simulink model "Main_Sim"  (R2018a)
settings: Solver=ode1  StartTime=0.0  StopTime=constants.t_end  FixedStep=constants.dt  RelTol=1e-3  EnableMultiTasking=on
settings Model: ExtModeTrigDuration=5000  Creator=bruders  LastModifiedBy=Joseph
settings SolverCC: PositivePriorityOrder=on
settings DataIOCC: LimitDataPoints=on  SaveFormat=Array
settings OptimizationCC: LifeSpan=inf
settings DebuggingCC: SolverPrmCheckMsg=warning  AllowSymbolicDim=off  SFUnexpectedBacktrackingDiag=warning  SFNoUnconditionalDefaultTransitionDiag=warning  SFExecutionAtInitializationDiag=none
settings HardwareCC: ProdBitPerPointer=32  ProdBitPerSizeT=32  ProdBitPerPtrDiffT=32  ProdLargestAtomicFloat=None  ProdIntDivRoundTo=Undefined  ProdEndianess=Unspecified  ProdWordSize=32  ProdHWDeviceType=32-bit Generic
settings ModelReferenceCC: PropagateSignalLabelsOutOfModel=off
settings RTWCC: Description=QUARC Win64 Target  SystemTargetFile=quarc_win64.tlc  TemplateMakefile=quarc_default_tmf
settings CodeAppCC: StateflowObjectComments=on
settings STFCustomTargetCC: TargetPreCompLibLocation=C:\PROGRA~3\QUARC\lib\2016b\win64\release  ConcurrentExecutionCompliant=on  GeneratePreprocessorConditionals=Disable all  SystemTargetFile=quarc_win64.tlc
settings GRTTargetCC: TargetPreCompLibLocation=C:\PROGRA~3\QUARC\lib\2016b\win64\release  TargetLangStandard=C89/C90 (ANSI)  ParMdlRefBuildCompliant=off  CompOptLevelCompliant=off  GeneratePreprocessorConditionals=Disable all  CombineOutputUpdateFcns=off  MatFileLogging=off  CPPClassGenCompliant=off  GRTInterface=on  UseToolchainInfoCompliant=off  ExtMode=on  ExtModeMexFile=quarc_comm
settings ConfigComp: CovMetricSettings=dw  CovHtmlReporting=on  CovSaveCumulativeToWorkspaceVar=on  CovSaveSingleToWorkspaceVar=on  CovExternalEMLEnable=off  CovSFcnEnable=off

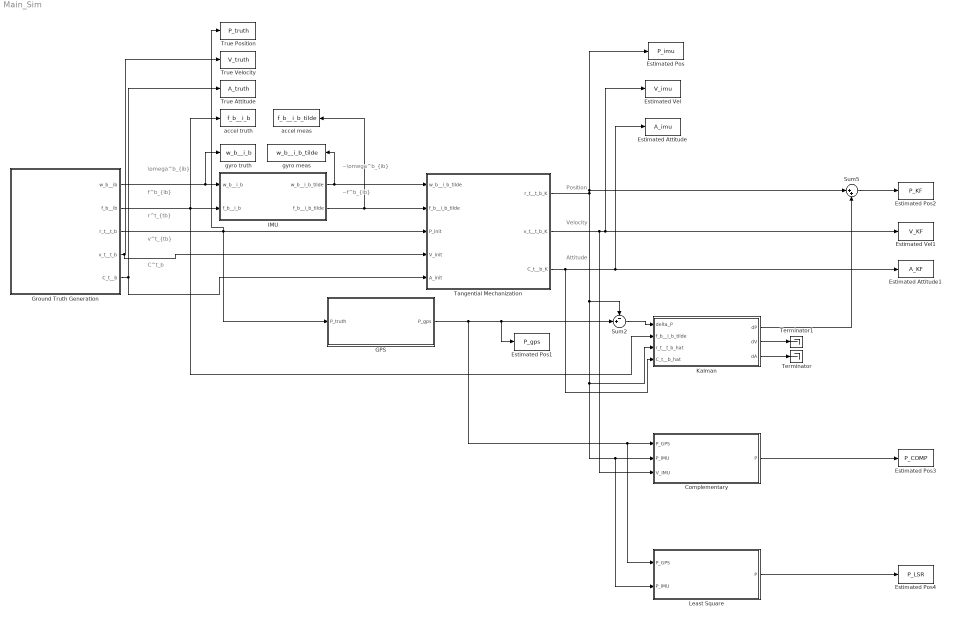
== system Main_Sim ==
  note: Position
  note: Velocity
  note: Attitude
  note: ~\omega^b_{ib}
  note: f^b_{ib}
  note: \omega^b_{ib}
  note: C^t_b
  note: ~f^b_{ib}
  note: v^t_{tb}
  note: r^t_{tb}
  Complementary : MATLAB Function  TreatAsAtomicUnit=on
  Estimated Attitude : ToWorkspace  VariableName=A_imu  SampleTime=-1
  Estimated Attitude1 : ToWorkspace  VariableName=A_KF  SampleTime=-1
  Estimated Pos : ToWorkspace  VariableName=P_imu  SampleTime=-1
  Estimated Pos1 : ToWorkspace  VariableName=P_gps  SampleTime=-1
  Estimated Pos2 : ToWorkspace  VariableName=P_KF  SampleTime=-1
  Estimated Pos3 : ToWorkspace  VariableName=P_COMP  SampleTime=-1
  Estimated Pos4 : ToWorkspace  VariableName=P_LSR  SampleTime=-1
  Estimated Vel : ToWorkspace  VariableName=V_imu  SampleTime=-1
  Estimated Vel1 : ToWorkspace  VariableName=V_KF  SampleTime=-1
  GPS : MATLAB Function  TreatAsAtomicUnit=on
  Ground Truth Generation : Subsystem
      mask Display: image('Gnd_truth.jpg');
  IMU : MATLAB Function  TreatAsAtomicUnit=on
  Kalman : MATLAB Function  TreatAsAtomicUnit=on
  Least Square : MATLAB Function  TreatAsAtomicUnit=on
  Sum2 : Sum  Inputs=-+|
  Sum5 : Sum  Inputs=|++
  Tangential Mechanization : MATLAB Function  TreatAsAtomicUnit=on
  Terminator : Terminator
  Terminator1 : Terminator
  True Attitude : ToWorkspace  VariableName=A_truth  SampleTime=-1
  True Position : ToWorkspace  VariableName=P_truth  SampleTime=-1
  True Velocity : ToWorkspace  VariableName=V_truth  SampleTime=-1
  accel meas : ToWorkspace  VariableName=f_b__i_b_tilde  SampleTime=-1
  accel truth : ToWorkspace  VariableName=f_b__i_b  SampleTime=-1
  gyro meas : ToWorkspace  VariableName=w_b__i_b_tilde  SampleTime=-1
  gyro truth : ToWorkspace  VariableName=w_b__i_b  SampleTime=-1
  wires:
  Tangential Mechanization/1(r_t__t_b_K) -> Sum5/1, Estimated Pos/1, Least Square/2(P_IMU), Complementary/2(P_IMU), Kalman/3(r_t__t_b_hat), Sum2/1
  Ground Truth Generation/1(w_b__ib) -> IMU/1(w_b__i_b), gyro truth/1
  Ground Truth Generation/2(f_b__ib) -> Kalman/2(f_b__i_b_tilde), IMU/2(f_b__i_b), accel truth/1
  Ground Truth Generation/3(r_t__t_b) -> Tangential Mechanization/3(P_init), GPS/1(P_truth), True Position/1
  Ground Truth Generation/4(v_t__t_b) -> Tangential Mechanization/4(V_init), True Velocity/1
  Ground Truth Generation/5(C_t__b) -> Tangential Mechanization/5(A_init), True Attitude/1
  IMU/1(w_b__i_b_tilde) -> Tangential Mechanization/1(w_b__i_b_tilde), gyro meas/1
  IMU/2(f_b__i_b_tilde) -> Tangential Mechanization/2(f_b__i_b_tilde), accel meas/1
  GPS/1(P_gps) -> Least Square/1(P_GPS), Complementary/1(P_GPS), Estimated Pos1/1, Sum2/2
  Sum2/1 -> Kalman/1(delta_P)
  Kalman/1(dP) -> Sum5/2
  Sum5/1 -> Estimated Pos2/1
  Tangential Mechanization/3(C_t__b_K) -> Kalman/4(C_t__b_hat), Estimated Attitude1/1, Estimated Attitude/1
  Kalman/3(dA) -> Terminator/1
  Tangential Mechanization/2(v_t__t_b_K) -> Complementary/3(V_IMU), Estimated Vel1/1, Estimated Vel/1
  Kalman/2(dV) -> Terminator1/1
  Complementary/1(P) -> Estimated Pos3/1
  Least Square/1(P) -> Estimated Pos4/1

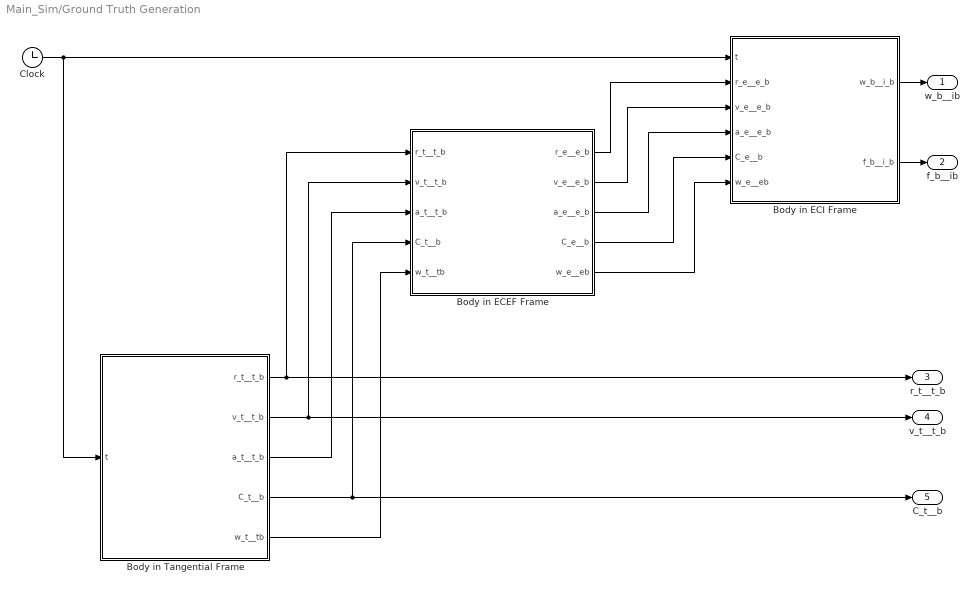
== system Main_Sim/Ground Truth Generation ==
  Body in ECEF Frame : MATLAB Function  TreatAsAtomicUnit=on
  Body in ECI Frame : MATLAB Function  TreatAsAtomicUnit=on
  Body in Tangential Frame : MATLAB Function  TreatAsAtomicUnit=on
  Clock : Clock
  w_b__ib : Outport  VectorParamsAs1DForOutWhenUnconnected=off
  f_b__ib : Outport  Port=2  VectorParamsAs1DForOutWhenUnconnected=off
  r_t__t_b : Outport  Port=3  VectorParamsAs1DForOutWhenUnconnected=off
  v_t__t_b : Outport  Port=4  VectorParamsAs1DForOutWhenUnconnected=off
  C_t__b : Outport  Port=5  VectorParamsAs1DForOutWhenUnconnected=off
  wires:
  Clock/1 -> Body in Tangential Frame/1(t), Body in ECI Frame/1(t)
  Body in Tangential Frame/1(r_t__t_b) -> Body in ECEF Frame/1(r_t__t_b), r_t__t_b/1
  Body in Tangential Frame/2(v_t__t_b) -> Body in ECEF Frame/2(v_t__t_b), v_t__t_b/1
  Body in Tangential Frame/4(C_t__b) -> C_t__b/1, Body in ECEF Frame/4(C_t__b)
  Body in Tangential Frame/3(a_t__t_b) -> Body in ECEF Frame/3(a_t__t_b)
  Body in ECEF Frame/1(r_e__e_b) -> Body in ECI Frame/2(r_e__e_b)
  Body in ECEF Frame/2(v_e__e_b) -> Body in ECI Frame/3(v_e__e_b)
  Body in ECEF Frame/3(a_e__e_b) -> Body in ECI Frame/4(a_e__e_b)
  Body in ECEF Frame/4(C_e__b) -> Body in ECI Frame/5(C_e__b)
  Body in Tangential Frame/5(w_t__tb) -> Body in ECEF Frame/5(w_t__tb)
  Body in ECI Frame/1(w_b__i_b) -> w_b__ib/1
  Body in ECEF Frame/5(w_e__eb) -> Body in ECI Frame/6(w_e__eb)
  Body in ECI Frame/2(f_b__i_b) -> f_b__ib/1

== matlab function Main_Sim/Ground Truth Generation/Body in ECEF Frame ==
  data: r_t__t_b input; v_t__t_b input; a_t__t_b input; C_t__b input; w_t__tb input; r_e__e_b output; constants parameter; v_e__e_b output; a_e__e_b output; C_e__b output; w_e__eb output
function [r_e__e_b, v_e__e_b, a_e__e_b, C_e__b, w_e__eb] = Tan_to_ECEF(r_t__t_b, v_t__t_b, a_t__t_b, C_t__b, w_t__tb, constants)
%#codegen
%
% FUNCTION DESCRIPTION:
%   Propagates quantities from the NAV to BODY coordinate frame
%
% INPUTS:
%   r_t__t_b = Position         of {b} wrt {t} resolved in {t} (m)
%   v_t__t_b = Velocity         of {b} wrt {t} resolved in {t} (m/s)
%   a_t__t_b = Acceleration     of {b} wrt {t} resolved in {t} (m/s^2)
%   C_t__b   = Attitude         of the b-frame wrt the t-frame
%   w_t__tb  = Angular Velocity of {b} wrt {t} resolved in {t} (rad/s)
%   constants= A structure containing various constant parameters
%
% OUTPUTS:
%   r_e__e_b = Position         of {b} wrt {e} resolved in {e} (m)
%   v_e__e_b = Velocity         of {b} wrt {e} resolved in {e} (m/s)
%   a_e__e_b = Acceleration     of {b} wrt {e} resolved in {e} (m/s^2)
%   C_e__b   = Attitude         of the b-frame wrt the e-frame
%   w_e__eb  = Angular Velocity of {b} wrt {e} resolved in {e} (rad/s)
%
% NOTES:
%   - None
%
% REFERENCE:
%   http://mercury.pr.erau.edu/~bruders EE 440 Modern Navigation

% Position of the t-frame wrt the e-frame resolved in {e} (m) - A constant vector
r_e__e_t = constants.r_e__e_t;

% Orientation/Attitude of the Tangential-frame wrt the ECEF-frame
C_e__t = constants.C_e__t ;

% Position of the b-frame wrt the e-frame resolved in {e} (m)
r_e__e_b = r_e__e_t + C_e__t * r_t__t_b;

% Velocity of the b-frame wrt the e-frame resolved in {e} (m/s)
v_e__e_b = C_e__t * v_t__t_b;
       
% Acceleration of the b-frame wrt the e-frame resolved in {e} (m/s^2)
a_e__e_b = C_e__t * a_t__t_b;
        
% Orientation/Attitude of the Body-frame wrt the ECEF-frame
 C_e__b = C_e__t * C_t__b;         

% Angular velocity of the b-frame wrt the e-frame resolved in {e} (rad/s)
w_e__eb = C_e__t * w_t__tb;

== matlab function Main_Sim/Complementary ==
  data: P_GPS input; P_IMU input; V_IMU input; constants parameter; P output
function P = Complementary(P_GPS, P_IMU, V_IMU, constants)
    persistent T
    % Keep track of the time
    if isempty(T)
        T = 0;
    else
        T = T + constants.dt;
    end
    alpha = T / constants.t_end;
    P = 0.5*P_GPS + 0.5*P_IMU;
end     % End of function

== matlab function Main_Sim/Ground Truth Generation/Body in ECI Frame ==
  data: t input; r_e__e_b input; v_e__e_b input; a_e__e_b input; C_e__b input; w_e__eb input; constants parameter; w_b__i_b output; f_b__i_b output
function [w_b__i_b, f_b__i_b] = ECEF_to_ECI(t, r_e__e_b, v_e__e_b, a_e__e_b, C_e__b, w_e__eb, constants)
%#codegen
%
% FUNCTION DESCRIPTION:
%   Propagates quantities from the NAV to BODY coordinate frame
%
% INPUTS:
%   r_e__e_b = Position         of {b} wrt {e} resolved in {e} (m)
%   v_e__e_b = Velocity         of {b} wrt {e} resolved in {e} (m/s)
%   a_e__e_b = Acceleration     of {b} wrt {e} resolved in {e} (m/s^2)
%   C_e__b   = Attitude         of the b-frame wrt the e-frame
%   w_e__eb  = Angular Velocity of {b} wrt {e} resolved in {e} (rad/s)
%   constants= A structure containing various constant parameters
%
% OUTPUTS:
%   w_i__i_b = Angular velocity of {b} wrt {i} resolved in {i} (rad/s)
%   a_i__i_b = Acceleration     of {b} wrt {i} resolved in {i} (m/s^2)
%
% NOTES:
%   - None
%
% REFERENCE:
%   http://mercury.pr.erau.edu/~bruders EE 440 Modern Navigation

w_i__i_e   = constants.w_i__i_e;            % Angular velocity of {e} wrt {i} resolved in {i} (rad/s)
Ohm_i__i_e = constants.Ohm_i__i_e;          % Skew symmetric version of w_i__i_e (rad/s)

% Generate Orientation (i.e., Attitude)
theta_e = constants.w_ie * t + 0;           % Rotational angle theta_e = w_ie t + theta_GMST

C_i__e = [ cos(theta_e), -sin(theta_e), 0   % Orientation of {e} wrt {i}
           sin(theta_e),  cos(theta_e), 0
           0           , 0            , 1];

% Position of the b-frame wrt the i-frame resolved in {i} (m)
r_i__i_b = C_i__e * r_e__e_b;

% Velocity of the b-frame wrt the i-frame resolved in {i} (m/s)
v_i__i_b = C_i__e * (v_e__e_b + Ohm_i__i_e * r_e__e_b);
       
% Acceleration of the b-frame wrt the i-frame resolved in {i} (m/s^2)
a_i__i_b = C_i__e * (a_e__e_b + 2*Ohm_i__i_e * v_e__e_b + Ohm_i__i_e * Ohm_i__i_e * r_e__e_b);
        
% Orientation/Attitude of the Body-frame wrt the ECI-frame
C_i__b = C_i__e * C_e__b;     

% Angular velocity: Ideal Gyro Measurements
w_b__i_b = C_i__b' * (w_i__i_e + C_i__e * w_e__eb);       % Ideal gyro measurements

% Specific Force: Ideal Accel Measurements
[L_b, lambda_b, h_b] = xyz2llh(r_e__e_b, constants);    % Compute the lat, lon, and height of body
g_n__b = [0; 0; gravity(L_b, h_b, constants)];          % Compute the acceleration due to gravity
C_e__n = Lat_Lon_2C_e__n(L_b, lambda_b);                % Compute C_e__n
g_e__b = C_e__n * g_n__b;                               % Compute the gravity of the body in the {e} frame
f_b__i_b = C_i__b' * (a_i__i_b - C_i__e * g_e__b - Ohm_i__i_e * Ohm_i__i_e * r_i__i_b);      % Ideal accel measurements

== matlab function Main_Sim/IMU ==
  data: w_b__i_b input; f_b__i_b input; constants parameter; w_b__i_b_tilde output; f_b__i_b_tilde output
function [w_b__i_b_tilde, f_b__i_b_tilde] = IMU(w_b__i_b, f_b__i_b, constants)
%#codegen
% FUNCTION DESCRIPTION:
%   Simulation of an IMU (ideal error-free case)
%
% INPUTS:
%   w_i__i_b = Angular velocity of {b} wrt {i} resolved in {i} (rad/s)
%   a_i__i_b = Acceleration     of {b} wrt {i} resolved in {i} (m/s^2)
%   constants= A structure containing many constant parameters
%
% OUTPUTS:
%   w_b__i_b_tilde = Gyro  meas (rad/s)
%   f_b__i_b_tilde = Accel meas (m/s^2)
%
% NOTES:
%   - None
%
% REFERENCE:
%   http://mercury.pr.erau.edu/~bruders EE 440 Modern Navigation

persistent b_g_BI b_a_BI                            % Persistent storage class variables

if isempty(b_g_BI)
    b_g_BI       = [0; 0; 0];                       % Initialize the Markov Bias Instability Bias term (rad/s)
    b_a_BI       = [0; 0; 0];                       % Initialize the Markov Bias Instability Bias term (m/s^2)     
end

dt           = constants.dt;    % Time step
I3           = eye(3);          % Identity matrix
Fs           = constants.Fs;    % Sample frequency
 % Gyro  related terms   
b_g_BI_sigma_n = constants.gyro.BI.sigma_n;         % Bias - White noise driving the Bias Instability 1-sigma (rad/s)

tau_g        = constants.gyro.BI.correlation_time;  % Correlation time for the bias instability (sec)
b_g_FB       = constants.gyro.b_g_FB;               % Bias - Fixed Bias term (rad/s)

sigma_ARW   = constants.gyro.sigma_ARW;             % Standard deviation of white noise due to ARW (rad/s)
M_g         = constants.gyro.M_g;                   % The combined Gyro Misalignment/Scale-Factor matrix
G_g         = constants.gyro.G_g;                   % The gyro G-sensitivity matrix (rad/sec/g)

 % Accel related terms   
b_a_BI_sigma_n = constants.accel.BI.sigma_n;        % Bias - White noise driving the Bias Instability 1-sigma (m/s^2)

tau_a        = constants.accel.BI.correlation_time; % Correlation time for the bias instability (sec)
b_a_FB       = constants.accel.b_a_FB;              % Bias - Fixed Bias term (m/s^2)

sigma_VRW   = constants.accel.sigma_VRW;            % Standard deviation of white noise due to VRW (m/s^2)
M_a         = constants.accel.M_a;                  % The combined Gyro Misalignment/Scale-Factor matrix    

%++++++++++++++++++++++++++++++++++++++++++++++++++++++++++++++++++++++++++
% Gyro Model:
%++++++++++++++++++++++++++++++++++++++++++++++++++++++++++++++++++++++++++

% Bias terms
b_g_BS = constants.gyro.b_g_BS;             % Bias - Bias Stability Bias term (rad/s)
b_g_BI = exp(-dt/tau_g) * b_g_BI + randn(3,1)*b_g_BI_sigma_n; % Bias - Markov Bias Instability Bias term (rad/s)
b_g = b_g_BI + b_g_FB + b_g_BS;             % All three bias terms (rad/s)

% Noise terms
w_g = sigma_ARW * randn(3,1);        % Gyro noise (rad/sec)

% Including all of the error terms
w_b__i_b_tilde = b_g + (I3 + M_g) * w_b__i_b + G_g * f_b__i_b + w_g;

%++++++++++++++++++++++++++++++++++++++++++++++++++++++++++++++++++++++++++
% Accelerometer Model
%++++++++++++++++++++++++++++++++++++++++++++++++++++++++++++++++++++++++++

% Bias terms
b_a_BS = constants.accel.b_a_BS;             % Bias - Bias Stability Bias term (m/s^2)
b_a_BI = exp(-dt/tau_a) * b_a_BI + randn(3,1)*b_a_BI_sigma_n; % Bias - Markov Bias Instability Bias term (m/s^2)
b_a = b_a_BI + b_a_FB + b_a_BS;             % All three bias terms (m/s^2)

% Noise terms
w_a = sigma_VRW * randn(3,1);        % Accelerometer noise (in m/s^2)

% Including all of the error terms
f_b__i_b_tilde = b_a + (I3 + M_a) * f_b__i_b + w_a;

== matlab function Main_Sim/Tangential Mechanization ==
  data: w_b__i_b_tilde input; r_t__t_b_K output; f_b__i_b_tilde input; P_init input; V_init input; A_init input; constants parameter; v_t__t_b_K output; C_t__b_K output
function [r_t__t_b_K, v_t__t_b_K, C_t__b_K] = TAN_mech(w_b__i_b_tilde, f_b__i_b_tilde, P_init, V_init, A_init, constants)
%#codegen
% FUNCTION DESCRIPTION:
%   Implements the low and high-fidelity Tangential Frame Mechanization
%
% INPUTS:
%   w_b__i_b_tilde  = Current Gyro measurements (rad/s)
%   f_b__i_b_tilde  = Current Accel measurements (m/s^2)
%   P_init          = True position r_t__t_b used to initialize (meters)
%   V_init          = True velocity v_t__t_b used to initialize (meters/sec)
%   A_init          = True attitude C_t__b used to initialize (dimless)
%
% OUTPUTS:
%   r_t__t_b_K      = Updated position r_t__t_b(k) = r_t__t_b(+) (meters)
%   v_t__t_b_K      = Updated velocity v_t__t_b(k) = v_t__t_b(+) (meters/sec)
%   C_t__b_K        = Updated attitude C_t__b(k)   = C_t__b(+)
%
%  Reference:  EE 440 Lecture notes:
%
%  NOTES:
%   1.) fidelity = 0 => Low-fidelity or = 1 => High-fidelity
%   2.) The True PVA is ONLY used to initialize the mechanization!!

persistent r_t__t_b_K_1 v_t__t_b_K_1 C_t__b_K_1

fidelity = constants.fidelity;      % Set to '0' for Low-fidelity and '1' for High-fidelity
dt       = constants.dt;            % Time step (sec)
I3       = eye(3);                  % 3X3 Identity matrix
Ohm_i__i_e = constants.Ohm_i__i_e;  % Earth Rate skew-symmetric matrix (rad/s)
w_i__i_e   = constants.w_i__i_e;    % Angular velocity of {e} wrt {i} resolved in {i} (rad/s)
C_e__t = constants.C_e__t;          % Attitude of t-frame wrt e-frame (a constant matrix)
C_t__e = C_e__t';
r_e__e_t = constants.r_e__e_t;      % Position of org of t-frame wrt e-frame resolved in e-frame

% If this is the first call to the function then Initialize the PVA
if isempty(C_t__b_K_1)      % Initialize the PVA (with zero for everything)
    r_t__t_b_K = P_init;
    v_t__t_b_K = V_init;
    C_t__b_K   = A_init;
    
    % Update PVA(k-1) = PVA(-) values
    r_t__t_b_K_1 = P_init; % Body and nav frame share common org
    v_t__t_b_K_1 = V_init;
    C_t__b_K_1   = A_init;
else
%==========================================================================
% Tangential Frame PVA Mechanization:
%==========================================================================
    Ohm_t__i_e = C_t__e * Ohm_i__i_e * C_e__t; % Earth rate in the t-frame
    
    %----------------------------------------------------------------------
    % STEP 1.) Attitude Update
    %----------------------------------------------------------------------    
    if ~fidelity                    % If "low-fidelity" eqns

    % First order approximation used (Lower fidelity eqns) ++++++++++++++++++++
    % Build skew-symmetric matrix Ohm from vector w
    Ohm_b__i_b_tilde = vec2ss(w_b__i_b_tilde); % (rad/s)
    %  t       t              b             t    t
    % C (k) = C (k-1) [I + Ohm (k) dt] - Ohm    C (k-1)
    %  b       b              ib            ie   b
    C_t__b_K = C_t__b_K_1 * (I3 + Ohm_b__i_b_tilde*dt) - Ohm_t__i_e * C_t__b_K_1*dt;

    else                            % If "high-fidelity" eqns
    % Higher fidelity equations +++++++++++++++++++++++++++++++++++++++++++++++
    %   t        t  b        t
    %  w  (k) = C  w  (k) - w 
    %   tb       b  ib       ie
    w_t__t_b = C_t__b_K_1 * w_b__i_b_tilde - C_t__e * w_i__i_e;  % (rad/s)
    %            t
    % Defining: w   dt = k d_theta, and K = Skew(k)
    %            tb
    
    %  t                                               2     t
    % C (k) = [I + sin(d_theta) K + (1 - cos(d_theta) K )]  C (k-1) 
    %  b                                                     b
    %
    C_t__b_K = Rodrigues_k(w_t__t_b*dt) * C_t__b_K_1; % 
    end
    
    %--------------------------------------------------------------------------
    % STEP 2.) Specific Force Update
    %----------------------------------------------------------------------
    %  t     t     b  
    % f   = C (k) f
    %  ib    b     ib
    f_t__i_b = C_t__b_K * f_b__i_b_tilde;   % (m/s^2)

    %--------------------------------------------------------------------------
    % STEP 3.) Velocity Update
    %----------------------------------------------------------------------
    % Gravity Calculation:
    % Since the body is above the ellipsoid use the "gravity" fn NOT Somigliana
    r_e__e_b = r_e__e_t + C_e__t * r_t__t_b_K_1;            % Compute r_e__e_b
    [L_b, lambda_b, h_b] = xyz2llh(r_e__e_b, constants);    % Compute the lat, lon, and height
    g_n__b = [0; 0; gravity(L_b, h_b, constants)];          % Compute the acceleration due to gravity
    C_e__n = Lat_Lon_2C_e__n(L_b, lambda_b);                % Compute C_e__n
    g_e__b = C_e__n * g_n__b;                               % Compute the gravity of the body in the {e} frame
    g_t__b = C_t__e * g_e__b;                               % Compute the gravity of the body in the {t} frame
    
    %  t    t     t        t   t
    % a  = f   + g  - 2 Ohm   v  (k-1)
    %  tb   ib    b        ie  tb
    a_t__t_b = f_t__i_b + g_t__b - 2*Ohm_t__i_e * v_t__t_b_K_1; % (m/s^2)

    %   t        t          t
    %  v  (k) = v  (k-1) + a   dt
    %   tb       tb         tb
    v_t__t_b_K = v_t__t_b_K_1 + a_t__t_b * dt;  % (m/s)

    %--------------------------------------------------------------------------
    % STEP 4.) Position Update
    %----------------------------------------------------------------------
    %   t        t          t             t         2
    %  r  (k) = r  (k-1) + v  (k-1) dt + a  (k-1) dt
    %   tb       tb         tb            tb
    r_t__t_b_K = r_t__t_b_K_1 + v_t__t_b_K_1*dt + a_t__t_b * dt^2 / 2; % slide 8 (m)
    
    % Store PVA(k-1) values for use in next iteration
    r_t__t_b_K_1 = r_t__t_b_K; % Body and nav frame share common org
    v_t__t_b_K_1 = v_t__t_b_K;
    C_t__b_K_1   = C_t__b_K;
end  % End of the t_sec == 0 block

end     % End of function

== matlab function Main_Sim/GPS ==
  data: P_truth input; constants parameter; P_gps output
function P_gps  = GPS(P_truth, constants)
%#codegen
% FUNCTION DESCRIPTION:
%   Simulation of an IMU (ideal error-free case)
%
% INPUTS:
%   w_i__i_b = Angular velocity of {b} wrt {i} resolved in {i} (rad/s)
%   a_i__i_b = Acceleration     of {b} wrt {i} resolved in {i} (m/s^2)
%   constants= A structure containing many constant parameters
%
% OUTPUTS:
%   w_b__i_b_tilde = Gyro  meas (rad/s)
%   f_b__i_b_tilde = Accel meas (m/s^2)
%
% NOTES:
%   - None
%
% REFERENCE:
%   http://mercury.pr.erau.edu/~bruders EE 440 Modern Navigation
% Take truth data and expand to measured GPS data

    sigma = constants.gps.sigma;                            % Radius of error
    P_error = normrnd(0,sigma,3,1);                % Error = radius of error * rand value
    P_gps = P_truth + P_error;                      % GPS = Truth + Error 
end

== matlab function Main_Sim/Ground Truth Generation/Body in Tangential Frame ==
  data: t input; r_t__t_b output; constants parameter; v_t__t_b output; a_t__t_b output; C_t__b output; w_t__tb output
function [r_t__t_b, v_t__t_b, a_t__t_b, C_t__b, w_t__tb] = Body_in_Tan(t, constants)
%#codegen
%
% FUNCTION DESCRIPTION:
%   Propagates quantities from the NAV to BODY coordinate frame
%
% INPUTS:
%   t_sec    = Time (sec)
%   constants= A structure containing various constant parameters
%
% OUTPUTS:
%   r_t__t_b = Position         of {b} wrt {t} resolved in {t} (m)
%   v_t__t_b = Velocity         of {b} wrt {t} resolved in {t} (m/s)
%   a_t__t_b = Acceleration     of {b} wrt {t} resolved in {t} (m/s^2)
%   C_t__b   = Attitude         of the b-frame wrt the t-frame (dimless)
%   w_t__tb  = Angular Velocity of {b} wrt {t} resolved in {t} (rad/s)
% NOTES:
%   - None
%
% REFERENCE:
%   http://mercury.pr.erau.edu/~bruders EE 440 Modern Navigation

persistent cnt C_t__bm

dT = constants.dt;                  % Sample interval (sec)

Tx = constants.t_end;               % Period of the figure eight (sec) 
fx = 1/Tx;                          % Freq of the Fig eight (Hz)
wx = 4*pi*fx;                       % Freq of the Fig eight (rad/s)

Ax = 20;                            % Amplitude of fig eight in x-dir
Ay = 100;                           % Amplitude of fig eight in y-dir
Az = 50;                            % Amplitude of fig eight in z-dir

% Position of the b-frame wrt the t-frame resolved in {t} (m)
r_t__t_b = [ Ax      * sin(wx*t)   % A North-East-Down (NED) frame
            -Ay      * sin((wx/2)*t)
            -Az      * sin((wx/4)*t)];

% Velocity of the b-frame wrt the t-frame resolved in {t} (m)
v_t__t_b = [ Ax*wx   * cos(wx*t)        % A North-East-Down (NED) frame
            -Ay*wx/2 * cos(t*wx/2)
            -Az*wx/4 * cos(t*wx/4)];  
       
% Accel of the org of the b-frame wrt the t-frame described in the t-frame
a_t__t_b = [-Ax*wx^2    * sin(wx*t)     % A North-East-Down (NED) frame
             Ay*wx^2/4  * sin(t*wx/2)
             Az*wx^2/16 * sin(t*wx/4)];       
        
% Orientation of the b-frame wrt the t-frame (a forward-right-down frame)
x_axis = v_t__t_b / norm(v_t__t_b);     % x-axis points "forward"
% See generic form of the RPY matrix
pitch = asin(-x_axis(3));               % pitch angle (rad)
roll  = 0;
yaw   = atan2(x_axis(2), x_axis(1));    % yaw angle (rad)
C_t__b = ypr2dcm(yaw, pitch, roll);

% Add some roll based on the y-axis accel in the body frame
a_temp = C_t__b' * a_t__t_b;
roll = atan2(a_temp(2), 10);            % Relative to ~g
C_t__b = ypr2dcm(yaw, pitch, roll);     % Update DCM        
 
if isempty(cnt) % First time into the function?
    w_t__tb = [0;0;0];  % Initialize at 0
    cnt = 1;            % Any value will do
    C_t__bm = eye(3);
else
    %% THis method of generating w from C has the undesired effect of
    %% causing the low-fidelity mech to be more accurate than the high!!!
    %% Change the way
%     C_t__b_dot = (C_t__b - C_t__bm)/dT; % C_dot
%     Ohm_t__tb = C_t__b_dot * C_t__b';   % OHM = C_dot C'
%     w_t__tb = ss2vec(Ohm_t__tb);        % OHM -> w
    Delta_C = C_t__b * C_t__bm';    % C_t__b(k) = exp(OHMC_t__tb*dT) C_t__b(k-1)
    w_t__tb = dcm2k(Delta_C) / dT;  % C_t__b(k) = C_t__b(k-1) exp(OHMC_b__tb*dT)
end
C_t__bm = C_t__b;   % Store the current DCM for use in the next iteration

== matlab function Main_Sim/Kalman ==
  data: delta_P input; f_b__i_b_tilde input; r_t__t_b_hat input; C_t__b_hat input; constants parameter; dP output; dV output; dA output
function [dP, dV, dA] = Kalman(delta_P, f_b__i_b_tilde, r_t__t_b_hat, C_t__b_hat, constants)
I3 = eye(3);
O3 = zeros(3);
sigma_gps = constants.gps.sigma;
dt         = constants.dt;          % Time step (sec)
Ohm_i__i_e = constants.Ohm_i__i_e;  % Skew symmetric version of w_i__i_e (rad/s)
C_e__t     = constants.C_e__t;   	% Attitude of t-frame wrt e-frame (a constant matrix)
C_t__e     = C_e__t';
r_e__e_t   = constants.r_e__e_t;    % Position of org of t-frame wrt e-frame resolved in e-frame
Df_b__i_b = constants.accel.BI.sigma_n;     % Assume error in accel is all BI
Dw_b__i_b = constants.gyro.BI.sigma_n;      % Assume error in gyro is all BI

persistent Delta_PVAk_1 P_k_1
   
if isempty(Delta_PVAk_1)    
    Delta_PVAk_1  = zeros(9,1);     % Initialize Delta_PVA(k-1)
    Delta_PVAk    = zeros(9,1);     % Initialize Delta_PVA(k-1)
    P_k_1         = 0.1 * eye(9);
    P_k           = 0.1 * eye(9);
else
%% Build the F matrix: See lecture 29 slide 7
    O3 = zeros(3,3);
% First row:
    Ohm_t__i_e = C_t__e * Ohm_i__i_e * C_e__t;  % Earth rate in the t-frame

% Second row:
    F21 = -vec2ss(C_t__b_hat * f_b__i_b_tilde); % Vector to Skew-Symmetric
  % Now build F23
    r_e__e_b_hat = r_e__e_t + C_e__t * r_t__t_b_hat;
    [L_b_hat, lambda_b_hat, h_b_hat] = xyz2llh(r_e__e_b_hat, constants);
    gamma_e__i_b = gamma__i_b(r_e__e_b_hat, constants);
    r_e__e_S = Geo_Radius(L_b_hat, constants);
 
    F23 = -C_t__e * 2 * gamma_e__i_b * r_e__e_b_hat' / (r_e__e_S * norm(r_e__e_b_hat)) * C_e__t;
     
    F = [ -Ohm_t__i_e   ,  O3               , O3
           F21          , -2* Ohm_t__i_e    , F23
           O3           ,  I3               , O3];

%% Build the B matrix: See lecture 29 slide 7
    B = [C_t__b_hat * Dw_b__i_b
         C_t__b_hat * Df_b__i_b
         O3];
%% Transform Eqns from continuous-time to discrete-time: Lecture 30 slides 9-10
    A = eye(9) + F*dt;                % Estimate of exp(F dt) = I + F dt + F^2 dt^2 /2! + ...
	Q = eye(9)*0.01;
    G  = (eye(9)*dt + F*dt^2/2) * B;    % Estimate of G = A^-1 (exp(F dt) - I ) B = (I dt + F dt^2 /2! + ...) B
    
    H = [I3, O3, O3];                   % Only have delta Position
    R = I3*sigma_gps;                       % R is based on the sigma of GPS
    [Delta_PVAk, P_k] = Kalman_Filter(Delta_PVAk_1, P_k_1, delta_P, A, H, Q, R, O3, O3);

    Delta_PVAk_1 = Delta_PVAk;
    P_k_1 = P_k;
end

    dP = Delta_PVAk(1:3,1);
    dV = Delta_PVAk(4:6,1);
    dA = Delta_PVAk(7:9,1);


end     % End of function

== matlab function Main_Sim/Least Square ==
  data: P_GPS input; P_IMU input; constants parameter; P output
function P = Least_Square(P_GPS, P_IMU , constants)
    % Basic Least Square filter implementation
    P = ((P_IMU./P_IMU.^2)+(P_GPS./P_GPS.^2))./((1./P_IMU.^2)+(1./P_GPS.^2));
end     % End of function
